simulink model "State_Space_Model"  (R2023a)
settings: Solver=VariableStepAuto  StartTime=0.0  StopTime=10  RelTol=1e-3
values from neighbouring files (symbols this model uses):
  A = [(2*s + 2), -(2*s + 1), -1 ... (first row only)    [mesh_analysis.m]
undefined symbols (not defined in the file or in its folder): B, C, D
settings Model: Creator=Michael Ali  LastModifiedBy=23350
settings DebuggingCC: UnconnectedInputMsg=warning  UnconnectedOutputMsg=warning  UnconnectedLineMsg=warning
settings ModelReferenceCC: EnableRefExpFcnMdlSchedulingChecks=on
settings RTWCC: DLArmComputeVersion=19.05

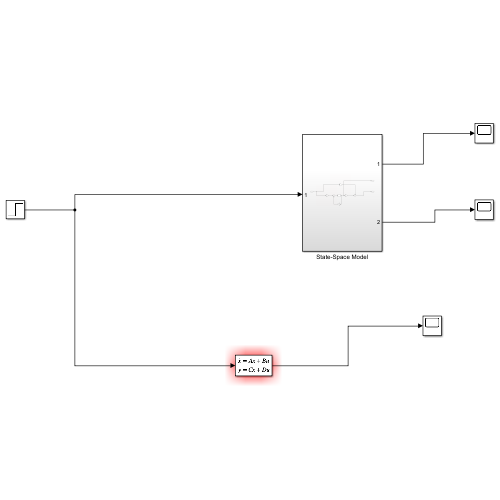
[thumbnail: Simulink's stored preview of the top-level diagram]
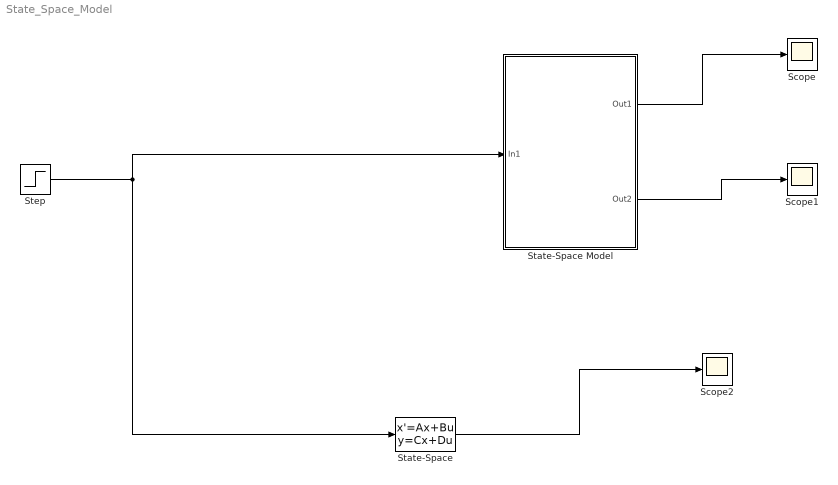
== system State_Space_Model ==
  Scope : Scope
  Scope1 : Scope
  Scope2 : Scope
  State-Space : StateSpace  A=A  B=B  C=C  D=D  InitialCondition=[1;0]
  State-Space Model : Subsystem
  Step : Step  SampleTime=0
  wires:
  State-Space/1 -> Scope2/1
  Step/1 -> State-Space/1, State-Space Model/1(In1)
  State-Space Model/1(Out1) -> Scope/1
  State-Space Model/2(Out2) -> Scope1/1

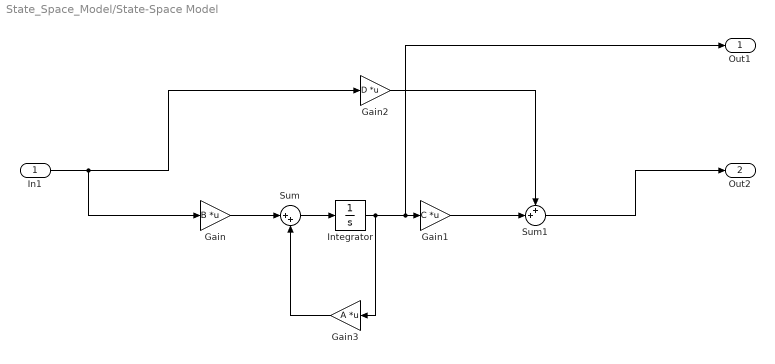
== system State_Space_Model/State-Space Model ==
  In1 : Inport
  Gain : Gain  Gain=B  Multiplication=Matrix(K*u)
  Gain1 : Gain  Gain=C  Multiplication=Matrix(K*u)
  Gain2 : Gain  Gain=D  Multiplication=Matrix(K*u)
  Gain3 : Gain  Gain=A  Multiplication=Matrix(K*u)
  Integrator : Integrator  InitialCondition=[1;0]
  Sum : Sum  Inputs=|++
  Sum1 : Sum  Inputs=++|
  Out1 : Outport
  Out2 : Outport  Port=2
  wires:
  Gain1/1 -> Sum1/2
  Gain2/1 -> Sum1/1
  Gain/1 -> Sum/1
  In1/1 -> Gain2/1, Gain/1
  Integrator/1 -> Out1/1, Gain1/1, Gain3/1
  Sum1/1 -> Out2/1
  Sum/1 -> Integrator/1
  Gain3/1 -> Sum/2
